simulink model "EH_agr_cluster"  (R2020a)
settings: Solver=VariableStepAuto  StartTime=0.0  StopTime=10.0  RelTol=1e-3
libraries: ODEHubs_components x21
settings Model: Creator=jero1  LastModifiedBy=jero1

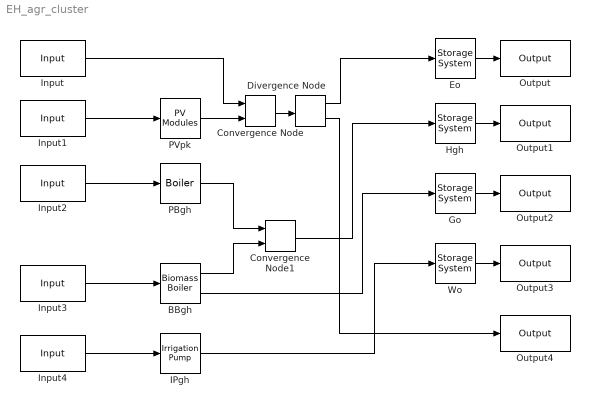
== system EH_agr_cluster ==
  BBgh : ODEHubs_components/Biomass Boiler  label=BBgh  n=2  nI=1:1  tI="\"B\""  nO=1:2  tO="[\"H\";\"G\"]"  sO=[1 1]  Dimin={1,1}  Dimax={40,40}  Domin={0,0}  Domax={inf,inf}  nd={4.25,1.76}
      settings: SourceProductName=ODEHubs
  Convergence Node : ODEHubs_components/Convergence Node  ID=CN1  n=1  Inputs=2
      settings: SourceProductName=ODEHubs
  Convergence Node1 : ODEHubs_components/Convergence Node  ID=CN2  n=2  Inputs=2
      settings: SourceProductName=ODEHubs
  Divergence Node : ODEHubs_components/Divergence Node  ID=DN1  n=1  Outputs=2
      settings: SourceProductName=ODEHubs
  Eo : ODEHubs_components/Storage System  label=Eo  n=1  Qchmin=0  Qchmax=3  nch=0.7  Qdismin=0  Qdismax=3  ndis=0.8  Smin=0  Smax=11  ns=0.98  S0=0
      settings: SourceProductName=ODEHubs
  Go : ODEHubs_components/Storage System  label=Go  n=3  Qchmin=0  Qchmax=51  nch=1  Qdismin=0  Qdismax=51  ndis=1  Smin=0  Smax=26.2  ns=1  S0=0
      settings: SourceProductName=ODEHubs
  Hgh : ODEHubs_components/Storage System  label=Hgh  n=2  Qchmin=0  Qchmax=104.5  nch=0.9  Qdismin=0  Qdismax=104.5  ndis=0.9  Smin=0  Smax=116.1  ns=0.94  S0=0
      settings: SourceProductName=ODEHubs
  IPgh : ODEHubs_components/Irrigation Pump  label=IPgh  n=1  nI=1:1  tI="\"W\""  nO=1:1  tO="\"W\""  sO=1  Dimin=0  Dimax=inf  Domin=0  Domax=5  nd=1
      settings: SourceProductName=ODEHubs
  Input : ODEHubs_components/Input  label=Ei  n=1  t=E  l='i'  colour=[0.6 0.6 0.6]  c='e_cost_func'  I_min=0  I_max=inf
      settings: SourceProductName=ODEHubs
  Input1 : ODEHubs_components/Input  label=Rpk  n=2  t=R  l='pk'  colour=[1 0.8 0]  c=0  I_min=0  I_max=inf
      settings: SourceProductName=ODEHubs
  Input2 : ODEHubs_components/Input  label=Pi  n=3  t=P  l='i'  colour=[1 0.6 1]  c=1.4*1.21  I_min=0  I_max=inf
      settings: SourceProductName=ODEHubs
  Input3 : ODEHubs_components/Input  label=Bi  n=4  t=B  l='i'  colour=[0.4 0.2 0.4]  c=0.255  I_min=0  I_max=inf
      settings: SourceProductName=ODEHubs
  Input4 : ODEHubs_components/Input  label=Wi  n=5  t=W  l='i'  colour=[0.4 1 0.4]  c=1.1*0.497  I_min=0  I_max=inf
      settings: SourceProductName=ODEHubs
  Output : ODEHubs_components/Output  label=Eo  n=1  t=E  l='o'  colour=[0.2 0.2 0.2]  dependance=none  prop=off  dev=0  devout=0  ms=off  f_label="{{\"Electric power (kW)\"}}"  st_label="{\"Stored energy (kWh)\"}"  factor=1.2  lb=0  ub=2  st_factor=1  st_lb=0  st_ub=2  O='Eo'  k=0  s='e_price_func'  M_min=0  M_max=inf
      settings: SourceProductName=ODEHubs
  Output1 : ODEHubs_components/Output  label=Hgh  n=2  t=H  l='gh'  colour=[0.6 0 0]  dependance=none  prop=off  dev=0  devout=0  ms=off  f_label="{{\"Thermal power  (kW)\"}}"  st_label="{\"Stored energy (kWh)\"}"  factor=1.2  lb=0  ub=16  st_factor=1  st_lb=0  st_ub=16  O='Hgh'  k=0  s=0  M_min=0  M_max=0
      settings: SourceProductName=ODEHubs
  Output2 : ODEHubs_components/Output  label=Go  n=3  t=G  l='o'  colour=[0.8 0.8 0.4]  dependance=none  prop=off  dev=0  devout=0  ms=on  f_label="{{\"Carbon dioxide (kg/h)\"}}"  st_label="{\"Stored mass (kg)\"}"  factor=1.2  lb=0  ub=8  st_factor=1  st_lb=0  st_ub=8  O='Go'  k=0  s=0  M_min=0  M_max=inf
      settings: SourceProductName=ODEHubs
  Output3 : ODEHubs_components/Output  label=Wo  n=4  t=W  l='o'  colour=[0 0.4 0]  dependance=none  prop=off  dev=0  devout=0  ms=off  f_label="{{\"Irrigation water (m^3/h)\"}}"  st_label="{\"Stored volume (m^3)\"}"  factor=1.2  lb=0  ub=2  st_factor=1  st_lb=0  st_ub=2  O='Wo'  k=0  s=0  M_min=0  M_max=0
      settings: SourceProductName=ODEHubs
  Output4 : ODEHubs_components/Output  label=Esgh  n=5  t=E  l='sgh'  colour=[0.2 0.2 0.2]  dependance=device  prop=off  dev=IPgh  devout=1  ms=off  f_label="{{\"Pump power (kW)\"}}"  st_label="{\" \"}"  factor=1.2  lb=0  ub=5  st_factor=1  st_lb=0  st_ub=5  O=4.5  k=0  s=0  M_min=0  M_max=0
      settings: SourceProductName=ODEHubs
  PBgh : ODEHubs_components/Boiler  label=PBgh  n=3  nI=1:1  tI="\"P\""  nO=1:1  tO="\"H\""  sO=1  Dimin=0  Dimax=6.8  Domin=0  Domax=inf  nd=11.54
      settings: SourceProductName=ODEHubs
  PVpk : ODEHubs_components/PV Modules  label=PVpk  n=4  nI=1:1  tI="\"R\""  nO=1:1  tO="\"E\""  sO=1  Dimin=0  Dimax='Dimax_pvpk_func'  Domin=0  Domax=inf  nd='npvpk_func'
      settings: SourceProductName=ODEHubs
  Wo : ODEHubs_components/Storage System  label=Wo  n=4  Qchmin=0  Qchmax=3  nch=1  Qdismin=0  Qdismax=3  ndis=1  Smin=0  Smax=6  ns=1  S0=0
      settings: SourceProductName=ODEHubs
  wires:
  Wo/1 -> Output3/1
  Go/1 -> Output2/1
  Hgh/1 -> Output1/1
  Eo/1 -> Output/1
  Input1/1 -> PVpk/1
  Input3/1 -> BBgh/1
  Input4/1 -> IPgh/1
  Input2/1 -> PBgh/1
  IPgh/1 -> Wo/1
  Input/1 -> Convergence Node/1
  PVpk/1 -> Convergence Node/2
  Convergence Node/1 -> Divergence Node/1
  Divergence Node/1 -> Eo/1
  Divergence Node/2 -> Output4/1
  BBgh/1 -> Convergence Node1/2
  PBgh/1 -> Convergence Node1/1
  Convergence Node1/1 -> Hgh/1
  BBgh/2 -> Go/1
